simulink model "model"  (R2014a)
(part 5 of 5)

  bus45 : powerlib/Measurements/Load Flow Bus  LConnTagsString=a  ID=bus45  Vbase=220000  Vref=1  Vangle=0  VLF=1  angleLF=0
      settings: AttributesFormatString=|
      | %<ID>
      | %<Vbase>V
      | %<VLF>pu
      | %<angleLF>deg.
      | %<Name>
  bus46 : powerlib/Measurements/Load Flow Bus  LConnTagsString=a  ID=bus46  Vbase=220000  Vref=1  Vangle=0  VLF=1  angleLF=0
      settings: AttributesFormatString=|
      | %<ID>
      | %<Vbase>V
      | %<VLF>pu
      | %<angleLF>deg.
      | %<Name>
  bus47 : powerlib/Measurements/Load Flow Bus  LConnTagsString=a  ID=bus47  Vbase=220000  Vref=1  Vangle=0  VLF=1  angleLF=0
      settings: AttributesFormatString=|
      | %<ID>
      | %<Vbase>V
      | %<VLF>pu
      | %<angleLF>deg.
      | %<Name>
  bus48 : powerlib/Measurements/Load Flow Bus  LConnTagsString=a  ID=bus48  Vbase=220000  Vref=1  Vangle=0  VLF=1  angleLF=0
      settings: AttributesFormatString=|
      | %<ID>
      | %<Vbase>V
      | %<VLF>pu
      | %<angleLF>deg.
      | %<Name>
  bus49 : powerlib/Measurements/Load Flow Bus  LConnTagsString=a  ID=bus49  Vbase=220000  Vref=1  Vangle=0  VLF=1  angleLF=0
      settings: AttributesFormatString=|
      | %<ID>
      | %<Vbase>V
      | %<VLF>pu
      | %<angleLF>deg.
      | %<Name>
  bus5 : powerlib/Measurements/Load Flow Bus  LConnTagsString=a  ID=bus5  Vbase=10000  Vref=1  Vangle=0  VLF=1  angleLF=0
      settings: AttributesFormatString=|
      | %<ID>
      | %<Vbase>V
      | %<VLF>pu
      | %<angleLF>deg.
      | %<Name>
  bus50 : powerlib/Measurements/Load Flow Bus  LConnTagsString=a  ID=bus50  Vbase=220000  Vref=1  Vangle=0  VLF=1  angleLF=0
      settings: AttributesFormatString=|
      | %<ID>
      | %<Vbase>V
      | %<VLF>pu
      | %<angleLF>deg.
      | %<Name>
  bus51 : powerlib/Measurements/Load Flow Bus  LConnTagsString=a  ID=bus51  Vbase=220000  Vref=1  Vangle=0  VLF=1  angleLF=0
      settings: AttributesFormatString=|
      | %<ID>
      | %<Vbase>V
      | %<VLF>pu
      | %<angleLF>deg.
      | %<Name>
  bus52 : powerlib/Measurements/Load Flow Bus  LConnTagsString=a  ID=bus52  Vbase=220000  Vref=1  Vangle=0  VLF=1  angleLF=0
      settings: AttributesFormatString=|
      | %<ID>
      | %<Vbase>V
      | %<VLF>pu
      | %<angleLF>deg.
      | %<Name>
  bus53 : powerlib/Measurements/Load Flow Bus  LConnTagsString=a  ID=bus53  Vbase=220000  Vref=1  Vangle=0  VLF=1  angleLF=0
      settings: AttributesFormatString=|
      | %<ID>
      | %<Vbase>V
      | %<VLF>pu
      | %<angleLF>deg.
      | %<Name>
  bus54 : powerlib/Measurements/Load Flow Bus  LConnTagsString=a  ID=bus54  Vbase=220000  Vref=1  Vangle=0  VLF=1  angleLF=0
      settings: AttributesFormatString=|
      | %<ID>
      | %<Vbase>V
      | %<VLF>pu
      | %<angleLF>deg.
      | %<Name>
  bus55 : powerlib/Measurements/Load Flow Bus  LConnTagsString=a  ID=bus55  Vbase=220000  Vref=1  Vangle=0  VLF=1  angleLF=0
      settings: AttributesFormatString=|
      | %<ID>
      | %<Vbase>V
      | %<VLF>pu
      | %<angleLF>deg.
      | %<Name>
  bus56 : powerlib/Measurements/Load Flow Bus  LConnTagsString=a  ID=bus56  Vbase=220000  Vref=1  Vangle=0  VLF=1  angleLF=0
      settings: AttributesFormatString=|
      | %<ID>
      | %<Vbase>V
      | %<VLF>pu
      | %<angleLF>deg.
      | %<Name>
  bus57 : powerlib/Measurements/Load Flow Bus  LConnTagsString=a  ID=bus57  Vbase=220000  Vref=1  Vangle=0  VLF=1  angleLF=0
      settings: AttributesFormatString=|
      | %<ID>
      | %<Vbase>V
      | %<VLF>pu
      | %<angleLF>deg.
      | %<Name>
  bus58 : powerlib/Measurements/Load Flow Bus  LConnTagsString=a  ID=bus58  Vbase=220000  Vref=1  Vangle=0  VLF=1  angleLF=0
      settings: AttributesFormatString=|
      | %<ID>
      | %<Vbase>V
      | %<VLF>pu
      | %<angleLF>deg.
      | %<Name>
  bus59 : powerlib/Measurements/Load Flow Bus  LConnTagsString=a  ID=bus59  Vbase=220000  Vref=1  Vangle=0  VLF=1  angleLF=0
      settings: AttributesFormatString=|
      | %<ID>
      | %<Vbase>V
      | %<VLF>pu
      | %<angleLF>deg.
      | %<Name>
  bus6 : powerlib/Measurements/Load Flow Bus  LConnTagsString=a  ID=bus6  Vbase=10000  Vref=1  Vangle=0  VLF=1  angleLF=0
      settings: AttributesFormatString=|
      | %<ID>
      | %<Vbase>V
      | %<VLF>pu
      | %<angleLF>deg.
      | %<Name>
  bus60 : powerlib/Measurements/Load Flow Bus  LConnTagsString=a  ID=bus60  Vbase=220000  Vref=1  Vangle=0  VLF=1  angleLF=0
      settings: AttributesFormatString=|
      | %<ID>
      | %<Vbase>V
      | %<VLF>pu
      | %<angleLF>deg.
      | %<Name>
  bus61 : powerlib/Measurements/Load Flow Bus  LConnTagsString=a  ID=bus61  Vbase=220000  Vref=1  Vangle=0  VLF=1  angleLF=0
      settings: AttributesFormatString=|
      | %<ID>
      | %<Vbase>V
      | %<VLF>pu
      | %<angleLF>deg.
      | %<Name>
  bus62 : powerlib/Measurements/Load Flow Bus  LConnTagsString=a  ID=bus62  Vbase=220000  Vref=1  Vangle=0  VLF=1  angleLF=0
      settings: AttributesFormatString=|
      | %<ID>
      | %<Vbase>V
      | %<VLF>pu
      | %<angleLF>deg.
      | %<Name>
  bus63 : powerlib/Measurements/Load Flow Bus  LConnTagsString=a  ID=bus63  Vbase=220000  Vref=1  Vangle=0  VLF=1  angleLF=0
      settings: AttributesFormatString=|
      | %<ID>
      | %<Vbase>V
      | %<VLF>pu
      | %<angleLF>deg.
      | %<Name>
  bus64 : powerlib/Measurements/Load Flow Bus  LConnTagsString=a  ID=bus64  Vbase=220000  Vref=1  Vangle=0  VLF=1  angleLF=0
      settings: AttributesFormatString=|
      | %<ID>
      | %<Vbase>V
      | %<VLF>pu
      | %<angleLF>deg.
      | %<Name>
  bus65 : powerlib/Measurements/Load Flow Bus  LConnTagsString=a  ID=bus65  Vbase=220000  Vref=1  Vangle=0  VLF=1  angleLF=0
      settings: AttributesFormatString=|
      | %<ID>
      | %<Vbase>V
      | %<VLF>pu
      | %<angleLF>deg.
      | %<Name>
  bus66 : powerlib/Measurements/Load Flow Bus  LConnTagsString=a  ID=bus66  Vbase=220000  Vref=1  Vangle=0  VLF=1  angleLF=0
      settings: AttributesFormatString=|
      | %<ID>
      | %<Vbase>V
      | %<VLF>pu
      | %<angleLF>deg.
      | %<Name>
  bus67 : powerlib/Measurements/Load Flow Bus  LConnTagsString=a  ID=bus67  Vbase=220000  Vref=1  Vangle=0  VLF=1  angleLF=0
      settings: AttributesFormatString=|
      | %<ID>
      | %<Vbase>V
      | %<VLF>pu
      | %<angleLF>deg.
      | %<Name>
  bus68 : powerlib/Measurements/Load Flow Bus  LConnTagsString=a  ID=bus68  Vbase=220000  Vref=1  Vangle=0  VLF=1  angleLF=0
      settings: AttributesFormatString=|
      | %<ID>
      | %<Vbase>V
      | %<VLF>pu
      | %<angleLF>deg.
      | %<Name>
  bus69 : powerlib/Measurements/Load Flow Bus  LConnTagsString=a  ID=bus69  Vbase=220000  Vref=1  Vangle=0  VLF=1  angleLF=0
      settings: AttributesFormatString=|
      | %<ID>
      | %<Vbase>V
      | %<VLF>pu
      | %<angleLF>deg.
      | %<Name>
  bus7 : powerlib/Measurements/Load Flow Bus  LConnTagsString=a  ID=bus7  Vbase=10000  Vref=1  Vangle=0  VLF=1  angleLF=0
      settings: AttributesFormatString=|
      | %<ID>
      | %<Vbase>V
      | %<VLF>pu
      | %<angleLF>deg.
      | %<Name>
  bus70 : powerlib/Measurements/Load Flow Bus  LConnTagsString=a  ID=bus70  Vbase=220000  Vref=1  Vangle=0  VLF=1  angleLF=0
      settings: AttributesFormatString=|
      | %<ID>
      | %<Vbase>V
      | %<VLF>pu
      | %<angleLF>deg.
      | %<Name>
  bus71 : powerlib/Measurements/Load Flow Bus  LConnTagsString=a  ID=bus71  Vbase=220000  Vref=1  Vangle=0  VLF=1  angleLF=0
      settings: AttributesFormatString=|
      | %<ID>
      | %<Vbase>V
      | %<VLF>pu
      | %<angleLF>deg.
      | %<Name>
  bus72 : powerlib/Measurements/Load Flow Bus  LConnTagsString=a  ID=bus72  Vbase=220000  Vref=1  Vangle=0  VLF=1  angleLF=0
      settings: AttributesFormatString=|
      | %<ID>
      | %<Vbase>V
      | %<VLF>pu
      | %<angleLF>deg.
      | %<Name>
  bus73 : powerlib/Measurements/Load Flow Bus  LConnTagsString=a  ID=bus73  Vbase=400000  Vref=1  Vangle=0  VLF=1  angleLF=0
      settings: AttributesFormatString=|
      | %<ID>
      | %<Vbase>V
      | %<VLF>pu
      | %<angleLF>deg.
      | %<Name>
  bus74 : powerlib/Measurements/Load Flow Bus  LConnTagsString=a  ID=bus74  Vbase=400000  Vref=1  Vangle=0  VLF=1  angleLF=0
      settings: AttributesFormatString=|
      | %<ID>
      | %<Vbase>V
      | %<VLF>pu
      | %<angleLF>deg.
      | %<Name>
  bus75 : powerlib/Measurements/Load Flow Bus  LConnTagsString=a  ID=bus75  Vbase=400000  Vref=1  Vangle=0  VLF=1  angleLF=0
      settings: AttributesFormatString=|
      | %<ID>
      | %<Vbase>V
      | %<VLF>pu
      | %<angleLF>deg.
      | %<Name>
  bus76 : powerlib/Measurements/Load Flow Bus  LConnTagsString=a  ID=bus76  Vbase=400000  Vref=1  Vangle=0  VLF=1  angleLF=0
      settings: AttributesFormatString=|
      | %<ID>
      | %<Vbase>V
      | %<VLF>pu
      | %<angleLF>deg.
      | %<Name>
  bus77 : powerlib/Measurements/Load Flow Bus  LConnTagsString=a  ID=bus77  Vbase=400000  Vref=1  Vangle=0  VLF=1  angleLF=0
      settings: AttributesFormatString=|
      | %<ID>
      | %<Vbase>V
      | %<VLF>pu
      | %<angleLF>deg.
      | %<Name>
  bus78 : powerlib/Measurements/Load Flow Bus  LConnTagsString=a  ID=bus78  Vbase=400000  Vref=1  Vangle=0  VLF=1  angleLF=0
      settings: AttributesFormatString=|
      | %<ID>
      | %<Vbase>V
      | %<VLF>pu
      | %<angleLF>deg.
      | %<Name>
  bus79 : powerlib/Measurements/Load Flow Bus  LConnTagsString=a  ID=bus79  Vbase=400000  Vref=1  Vangle=0  VLF=1  angleLF=0
      settings: AttributesFormatString=|
      | %<ID>
      | %<Vbase>V
      | %<VLF>pu
      | %<angleLF>deg.
      | %<Name>
  bus8 : powerlib/Measurements/Load Flow Bus  LConnTagsString=a  ID=bus8  Vbase=10000  Vref=1  Vangle=0  VLF=1  angleLF=0
      settings: AttributesFormatString=|
      | %<ID>
      | %<Vbase>V
      | %<VLF>pu
      | %<angleLF>deg.
      | %<Name>
  bus80 : powerlib/Measurements/Load Flow Bus  LConnTagsString=a  ID=bus80  Vbase=400000  Vref=1  Vangle=0  VLF=1  angleLF=0
      settings: AttributesFormatString=|
      | %<ID>
      | %<Vbase>V
      | %<VLF>pu
      | %<angleLF>deg.
      | %<Name>
  bus81 : powerlib/Measurements/Load Flow Bus  LConnTagsString=a  ID=bus81  Vbase=400000  Vref=1  Vangle=0  VLF=1  angleLF=0
      settings: AttributesFormatString=|
      | %<ID>
      | %<Vbase>V
      | %<VLF>pu
      | %<angleLF>deg.
      | %<Name>
  bus82 : powerlib/Measurements/Load Flow Bus  LConnTagsString=a  ID=bus82  Vbase=400000  Vref=1  Vangle=0  VLF=1  angleLF=0
      settings: AttributesFormatString=|
      | %<ID>
      | %<Vbase>V
      | %<VLF>pu
      | %<angleLF>deg.
      | %<Name>
  bus83 : powerlib/Measurements/Load Flow Bus  LConnTagsString=a  ID=bus83  Vbase=400000  Vref=1  Vangle=0  VLF=1  angleLF=0
      settings: AttributesFormatString=|
      | %<ID>
      | %<Vbase>V
      | %<VLF>pu
      | %<angleLF>deg.
      | %<Name>
  bus84 : powerlib/Measurements/Load Flow Bus  LConnTagsString=a  ID=bus84  Vbase=400000  Vref=1  Vangle=0  VLF=1  angleLF=0
      settings: AttributesFormatString=|
      | %<ID>
      | %<Vbase>V
      | %<VLF>pu
      | %<angleLF>deg.
      | %<Name>
  bus85 : powerlib/Measurements/Load Flow Bus  LConnTagsString=a  ID=bus85  Vbase=400000  Vref=1  Vangle=0  VLF=1  angleLF=0
      settings: AttributesFormatString=|
      | %<ID>
      | %<Vbase>V
      | %<VLF>pu
      | %<angleLF>deg.
      | %<Name>
  bus86 : powerlib/Measurements/Load Flow Bus  LConnTagsString=a  ID=bus86  Vbase=400000  Vref=1  Vangle=0  VLF=1  angleLF=0
      settings: AttributesFormatString=|
      | %<ID>
      | %<Vbase>V
      | %<VLF>pu
      | %<angleLF>deg.
      | %<Name>
  bus87 : powerlib/Measurements/Load Flow Bus  LConnTagsString=a  ID=bus87  Vbase=400000  Vref=1  Vangle=0  VLF=1  angleLF=0
      settings: AttributesFormatString=|
      | %<ID>
      | %<Vbase>V
      | %<VLF>pu
      | %<angleLF>deg.
      | %<Name>
  bus88 : powerlib/Measurements/Load Flow Bus  LConnTagsString=a  ID=bus88  Vbase=400000  Vref=1  Vangle=0  VLF=1  angleLF=0
      settings: AttributesFormatString=|
      | %<ID>
      | %<Vbase>V
      | %<VLF>pu
      | %<angleLF>deg.
      | %<Name>
  bus89 : powerlib/Measurements/Load Flow Bus  LConnTagsString=a  ID=bus89  Vbase=400000  Vref=1  Vangle=0  VLF=1  angleLF=0
      settings: AttributesFormatString=|
      | %<ID>
      | %<Vbase>V
      | %<VLF>pu
      | %<angleLF>deg.
      | %<Name>
  bus9 : powerlib/Measurements/Load Flow Bus  LConnTagsString=a  ID=bus9  Vbase=10000  Vref=1  Vangle=0  VLF=1  angleLF=0
      settings: AttributesFormatString=|
      | %<ID>
      | %<Vbase>V
      | %<VLF>pu
      | %<angleLF>deg.
      | %<Name>
  bus90 : powerlib/Measurements/Load Flow Bus  LConnTagsString=a  ID=bus90  Vbase=400000  Vref=1  Vangle=0  VLF=1  angleLF=0
      settings: AttributesFormatString=|
      | %<ID>
      | %<Vbase>V
      | %<VLF>pu
      | %<angleLF>deg.
      | %<Name>
  bus91 : powerlib/Measurements/Load Flow Bus  LConnTagsString=a  ID=bus91  Vbase=400000  Vref=1  Vangle=0  VLF=1  angleLF=0
      settings: AttributesFormatString=|
      | %<ID>
      | %<Vbase>V
      | %<VLF>pu
      | %<angleLF>deg.
      | %<Name>
  bus92 : powerlib/Measurements/Load Flow Bus  LConnTagsString=a  ID=bus92  Vbase=400000  Vref=1  Vangle=0  VLF=1  angleLF=0
      settings: AttributesFormatString=|
      | %<ID>
      | %<Vbase>V
      | %<VLF>pu
      | %<angleLF>deg.
      | %<Name>
  bus93 : powerlib/Measurements/Load Flow Bus  LConnTagsString=a  ID=bus93  Vbase=400000  Vref=1  Vangle=0  VLF=1  angleLF=0
      settings: AttributesFormatString=|
      | %<ID>
      | %<Vbase>V
      | %<VLF>pu
      | %<angleLF>deg.
      | %<Name>
  bus94 : powerlib/Measurements/Load Flow Bus  LConnTagsString=a  ID=bus94  Vbase=400000  Vref=1  Vangle=0  VLF=1  angleLF=0
      settings: AttributesFormatString=|
      | %<ID>
      | %<Vbase>V
      | %<VLF>pu
      | %<angleLF>deg.
      | %<Name>
  bus95 : powerlib/Measurements/Load Flow Bus  LConnTagsString=a  ID=bus95  Vbase=400000  Vref=1  Vangle=0  VLF=1  angleLF=0
      settings: AttributesFormatString=|
      | %<ID>
      | %<Vbase>V
      | %<VLF>pu
      | %<angleLF>deg.
      | %<Name>
  bus96 : powerlib/Measurements/Load Flow Bus  LConnTagsString=a  ID=bus96  Vbase=400000  Vref=1  Vangle=0  VLF=1  angleLF=0
      settings: AttributesFormatString=|
      | %<ID>
      | %<Vbase>V
      | %<VLF>pu
      | %<angleLF>deg.
      | %<Name>
  bus97 : powerlib/Measurements/Load Flow Bus  LConnTagsString=a  ID=bus97  Vbase=400000  Vref=1  Vangle=0  VLF=1  angleLF=0
      settings: AttributesFormatString=|
      | %<ID>
      | %<Vbase>V
      | %<VLF>pu
      | %<angleLF>deg.
      | %<Name>
  bus98 : powerlib/Measurements/Load Flow Bus  LConnTagsString=a  ID=bus98  Vbase=400000  Vref=1  Vangle=0  VLF=1  angleLF=0
      settings: AttributesFormatString=|
      | %<ID>
      | %<Vbase>V
      | %<VLF>pu
      | %<angleLF>deg.
      | %<Name>
  bus99 : powerlib/Measurements/Load Flow Bus  LConnTagsString=a  ID=bus99  Vbase=400000  Vref=1  Vangle=0  VLF=1  angleLF=0
      settings: AttributesFormatString=|
      | %<ID>
      | %<Vbase>V
      | %<VLF>pu
      | %<angleLF>deg.
      | %<Name>
  powergui : powerlib/powergui  Priority=1  SimulationMode=Continuous  SolverType=Tustin  SampleTime=50e-6  frequency=60  SPID=off  DisableSnubberDevices=off  DisableRonSwitches=off  DisableVfSwitches=off  SwTol=0  Interpol=off  DisplayEquations=off  Ts=0  methode=off  frequencyindice=60  Pbase=100e6  ErrMax=1e-4  Iterations=50  UnitsV=kV  UnitsW=MW  FunctionMessages=off  echomessages=off  HookPort=off  EnableUseOfTLC=off  x0status=blocks  RestoreLinks=warning  ResistiveCurrentMeasurement=off  Frange=[0:2:500]  Ylog=off  Xlog=on  ShowGrid=off  save=off  variable=ZData  structure=0  ZoomFFT=off  StartTime=0.0  cycles=1  DisplayStyle=1  fundamental=60  FreqAxis=off  MaxFrequency=1000  frequencyindicesteady=1  RmsSteady=1  display=off
  Ötztal___Zirl_CN_147563007_110000_CN_100404264_110000 : powerlib/Elements/Distributed Parameters Line  Phases=3  Frequency=60  Resistance=[0.01273 0.3864]  Inductance="[0.9337e-3  4.1264e-3]"  Capacitance=[12.74e-9 7.751e-9]  Length=100  x1=[0 0 0 0; 0.0001244 0 0 0; 0.0002488 0 0 0; 0.0003733 0 0 0; 0.0004977 0 0 0; 0.0006221 0 0 0]  x2=[0 0 0 0; 0.0001244 0 0 0; 0.0002488 0 0 0; 0.0003733 0 0 0; 0.0004977 0 0 0; 0.0006221 0 0 0]  x3=[0 0 0 0; 0.0001244 0 0 0; 0.0002488 0 0 0; 0.0003733 0 0 0; 0.0004977 0 0 0; 0.0006221 0 0 0]  x4=[0 0 0 0; 0.0001244 0 0 0; 0.0002488 0 0 0; 0.0003733 0 0 0; 0.0004977 0 0 0; 0.0006221 0 0 0]  x5=0  V1=ones(3,3)  V2=ones(3,3)  I1=ones(3,3)  I2=ones(3,3)  nHarmo=1  Measurements=None
  connections:
  T_48374400__/LConn1 -- _CN_48374400_10000_CN_46584322_10000/LConn1
  T_48374400__/LConn2 -- _CN_48374400_10000_CN_46584322_10000/LConn2
  _CN_48374400_10000_CN_46584322_10000/LConn3 -- T_48374400__/LConn3 -- bus1/LConn1
  T_46584322__/LConn1 -- _CN_48374400_10000_CN_46584322_10000/RConn1
  T_46584322__/LConn2 -- _CN_48374400_10000_CN_46584322_10000/RConn2
  _CN_48374400_10000_CN_46584322_10000/RConn3 -- T_46584322__/LConn3 -- bus2/LConn1
  _CN_209067396_10000_CN_30621843_10000/LConn1 -- T_209067396__/LConn1 -- _CN_209067396_10000_CN_30622639_10000/LConn1
  _CN_209067396_10000_CN_30621843_10000/LConn2 -- T_209067396__/LConn2 -- _CN_209067396_10000_CN_30622639_10000/LConn2
  _CN_209067396_10000_CN_30621843_10000/LConn3 -- T_209067396__/LConn3 -- _CN_209067396_10000_CN_30622639_10000/LConn3 -- bus3/LConn1
  T_30621843__/LConn1 -- _CN_209067396_10000_CN_30621843_10000/RConn1
  T_30621843__/LConn2 -- _CN_209067396_10000_CN_30621843_10000/RConn2
  _CN_209067396_10000_CN_30621843_10000/RConn3 -- T_30621843__/LConn3 -- bus4/LConn1
  _CN_209067396_10000_CN_30622639_10000/RConn1 -- T_30622639__/LConn1 -- _CN_30622639_10000_CN_37036252_10000/LConn1
  _CN_209067396_10000_CN_30622639_10000/RConn2 -- T_30622639__/LConn2 -- _CN_30622639_10000_CN_37036252_10000/LConn2
  _CN_209067396_10000_CN_30622639_10000/RConn3 -- T_30622639__/LConn3 -- _CN_30622639_10000_CN_37036252_10000/LConn3 -- bus5/LConn1
  T_207939980__/LConn1 -- 110kV_CN_207939980_10000_CN_97334781_10000/LConn1
  T_207939980__/LConn2 -- 110kV_CN_207939980_10000_CN_97334781_10000/LConn2
  110kV_CN_207939980_10000_CN_97334781_10000/LConn3 -- T_207939980__/LConn3 -- bus6/LConn1
  110kV_CN_207939980_10000_CN_97334781_10000/RConn1 -- T_97334781__/RConn1 -- _CN_97334822_10000_CN_97334781_10000/LConn1 -- _CN_97418808_10000_CN_97334781_10000/LConn1 -- _CN_176828096_10000_CN_97334781_10000/LConn1 -- L_97334781/LConn1 -- 110kV_CN_176819478_10000_CN_97334781_10000/LConn1
  110kV_CN_207939980_10000_CN_97334781_10000/RConn2 -- T_97334781__/RConn2 -- _CN_97334822_10000_CN_97334781_10000/LConn2 -- _CN_97418808_10000_CN_97334781_10000/LConn2 -- _CN_176828096_10000_CN_97334781_10000/LConn2 -- L_97334781/LConn2 -- 110kV_CN_176819478_10000_CN_97334781_10000/LConn2
  110kV_CN_207939980_10000_CN_97334781_10000/RConn3 -- T_97334781__/RConn3 -- _CN_97334822_10000_CN_97334781_10000/LConn3 -- _CN_97418808_10000_CN_97334781_10000/LConn3 -- _CN_176828096_10000_CN_97334781_10000/LConn3 -- L_97334781/LConn3 -- bus7/LConn1 -- 110kV_CN_176819478_10000_CN_97334781_10000/LConn3
  T_176819478__Statie_de_transformare_110kV_20kV/LConn1 -- 110kV_CN_176819478_10000_CN_97334781_10000/RConn1
  T_176819478__Statie_de_transformare_110kV_20kV/LConn2 -- 110kV_CN_176819478_10000_CN_97334781_10000/RConn2
  110kV_CN_176819478_10000_CN_97334781_10000/RConn3 -- T_176819478__Statie_de_transformare_110kV_20kV/LConn3 -- bus8/LConn1
  _CN_234876695_10000_CN_97418808_10000/LConn1 -- T_234876695__/RConn4 -- L_234876695/LConn1
  _CN_234876695_10000_CN_97418808_10000/LConn2 -- T_234876695__/RConn5 -- L_234876695/LConn2
  _CN_234876695_10000_CN_97418808_10000/LConn3 -- T_234876695__/RConn6 -- L_234876695/LConn3 -- bus9/LConn1
  _CN_234876695_10000_CN_97418808_10000/RConn1 -- T_97418808__/LConn1 -- _CN_97418808_10000_CN_97334781_10000/RConn1
  _CN_234876695_10000_CN_97418808_10000/RConn2 -- T_97418808__/LConn2 -- _CN_97418808_10000_CN_97334781_10000/RConn2
  _CN_234876695_10000_CN_97418808_10000/RConn3 -- T_97418808__/LConn3 -- _CN_97418808_10000_CN_97334781_10000/RConn3 -- bus10/LConn1
  T_204932122__/LConn1 -- _CN_204932122_10000_CN_198333274_10000/LConn1
  T_204932122__/LConn2 -- _CN_204932122_10000_CN_198333274_10000/LConn2
  _CN_204932122_10000_CN_198333274_10000/LConn3 -- T_204932122__/LConn3 -- bus11/LConn1
  T_198333274__/LConn1 -- _CN_204932122_10000_CN_198333274_10000/RConn1
  T_198333274__/LConn2 -- _CN_204932122_10000_CN_198333274_10000/RConn2
  _CN_204932122_10000_CN_198333274_10000/RConn3 -- T_198333274__/LConn3 -- bus12/LConn1
  T_97334822__/LConn1 -- _CN_97334822_10000_CN_97334781_10000/RConn1
  T_97334822__/LConn2 -- _CN_97334822_10000_CN_97334781_10000/RConn2
  _CN_97334822_10000_CN_97334781_10000/RConn3 -- T_97334822__/LConn3 -- bus13/LConn1
  _CN_28251692_10000_CN_30618879_10000/LConn1 -- T_28251692__/RConn1 -- L_28251692/LConn1
  _CN_28251692_10000_CN_30618879_10000/LConn2 -- T_28251692__/RConn2 -- L_28251692/LConn2
  _CN_28251692_10000_CN_30618879_10000/LConn3 -- T_28251692__/RConn3 -- L_28251692/LConn3 -- bus14/LConn1
  G_30618879_CET_Vest/RConn1 -- _CN_28251692_10000_CN_30618879_10000/RConn1
  G_30618879_CET_Vest/RConn2 -- _CN_28251692_10000_CN_30618879_10000/RConn2
  _CN_28251692_10000_CN_30618879_10000/RConn3 -- G_30618879_CET_Vest/RConn3 -- bus15/LConn1
  _CN_30622639_10000_CN_37036252_10000/RConn1 -- T_37036252__/LConn1 -- _CN_37036252_10000_CN_29975403_10000/LConn1
  _CN_30622639_10000_CN_37036252_10000/RConn2 -- T_37036252__/LConn2 -- _CN_37036252_10000_CN_29975403_10000/LConn2
  _CN_30622639_10000_CN_37036252_10000/RConn3 -- T_37036252__/LConn3 -- _CN_37036252_10000_CN_29975403_10000/LConn3 -- bus16/LConn1
  _CN_176828096_10000_CN_97334781_10000/RConn1 -- T_176828096__/LConn1 -- _CN_176828096_10000_CN_235313249_10000/LConn1
  _CN_176828096_10000_CN_97334781_10000/RConn2 -- T_176828096__/LConn2 -- _CN_176828096_10000_CN_235313249_10000/LConn2
  _CN_176828096_10000_CN_97334781_10000/RConn3 -- T_176828096__/LConn3 -- _CN_176828096_10000_CN_235313249_10000/LConn3 -- bus17/LConn1
  T_235313249__/LConn1 -- _CN_176828096_10000_CN_235313249_10000/RConn1
  T_235313249__/LConn2 -- _CN_176828096_10000_CN_235313249_10000/RConn2
  _CN_176828096_10000_CN_235313249_10000/RConn3 -- T_235313249__/LConn3 -- bus18/LConn1
  T_29975403__/LConn1 -- _CN_37036252_10000_CN_29975403_10000/RConn1
  T_29975403__/LConn2 -- _CN_37036252_10000_CN_29975403_10000/RConn2
  _CN_37036252_10000_CN_29975403_10000/RConn3 -- T_29975403__/LConn3 -- bus19/LConn1
  T_89071477__/LConn1 -- _CN_89071477_10000_CN_46269303_10000/LConn1
  T_89071477__/LConn2 -- _CN_89071477_10000_CN_46269303_10000/LConn2
  _CN_89071477_10000_CN_46269303_10000/LConn3 -- T_89071477__/LConn3 -- bus20/LConn1
  T_46269303__/LConn1 -- _CN_89071477_10000_CN_46269303_10000/RConn1
  T_46269303__/LConn2 -- _CN_89071477_10000_CN_46269303_10000/RConn2
  _CN_89071477_10000_CN_46269303_10000/RConn3 -- T_46269303__/LConn3 -- bus21/LConn1
  T_278910976__/LConn1 -- _CN_278910976_220000_CN_199657993_220000/LConn1
  T_278910976__/LConn2 -- _CN_278910976_220000_CN_199657993_220000/LConn2
  _CN_278910976_220000_CN_199657993_220000/LConn3 -- T_278910976__/LConn3 -- bus22/LConn1
  T_199657993__/LConn1 -- _CN_278910976_220000_CN_199657993_220000/RConn1
  T_199657993__/LConn2 -- _CN_278910976_220000_CN_199657993_220000/RConn2
  _CN_278910976_220000_CN_199657993_220000/RConn3 -- T_199657993__/LConn3 -- bus23/LConn1
  T_208744453__/LConn1 -- _CN_208744453_220000_CN_228718321_220000/LConn1
  T_208744453__/LConn2 -- _CN_208744453_220000_CN_228718321_220000/LConn2
  _CN_208744453_220000_CN_228718321_220000/LConn3 -- T_208744453__/LConn3 -- bus24/LConn1
  _CN_208744453_220000_CN_228718321_220000/RConn1 -- T_228718321__/RConn1 -- _CN_208263464_220000_CN_228718321_220000/LConn1 -- L_228718321/LConn1
  _CN_208744453_220000_CN_228718321_220000/RConn2 -- T_228718321__/RConn2 -- _CN_208263464_220000_CN_228718321_220000/LConn2 -- L_228718321/LConn2
  _CN_208744453_220000_CN_228718321_220000/RConn3 -- T_228718321__/RConn3 -- _CN_208263464_220000_CN_228718321_220000/LConn3 -- L_228718321/LConn3 -- bus25/LConn1
  T_198276673__/LConn1 -- _CN_198276673_220000_CN_202461729_220000/LConn1
  T_198276673__/LConn2 -- _CN_198276673_220000_CN_202461729_220000/LConn2
  _CN_198276673_220000_CN_202461729_220000/LConn3 -- T_198276673__/LConn3 -- bus26/LConn1
  _CN_198276673_220000_CN_202461729_220000/RConn1 -- T_202461729__/LConn1 -- _CN_202948507_220000_CN_202461729_220000/LConn1
  _CN_198276673_220000_CN_202461729_220000/RConn2 -- T_202461729__/LConn2 -- _CN_202948507_220000_CN_202461729_220000/LConn2
  _CN_198276673_220000_CN_202461729_220000/RConn3 -- T_202461729__/LConn3 -- _CN_202948507_220000_CN_202461729_220000/LConn3 -- bus27/LConn1
  _CN_98111242_220000_CN_196654384_220000/LConn1 -- T_98111242__/LConn1 -- _CN_98111242_220000_CN_208263479_220000/LConn1 -- _CN_98111242_220000_CN_198283094_220000/LConn1 -- _CN_98111242_220000_CN_234876695_220000/LConn1 -- _CN_98111242_220000_CN_196654364_220000/LConn1 -- _CN_98111242_220000_CN_196654362_220000/LConn1 -- _CN_98111242_220000_CN_88174437_220000/LConn1
  _CN_98111242_220000_CN_196654384_220000/LConn2 -- T_98111242__/LConn2 -- _CN_98111242_220000_CN_208263479_220000/LConn2 -- _CN_98111242_220000_CN_198283094_220000/LConn2 -- _CN_98111242_220000_CN_234876695_220000/LConn2 -- _CN_98111242_220000_CN_196654364_220000/LConn2 -- _CN_98111242_220000_CN_196654362_220000/LConn2 -- _CN_98111242_220000_CN_88174437_220000/LConn2
  _CN_98111242_220000_CN_196654384_220000/LConn3 -- T_98111242__/LConn3 -- _CN_98111242_220000_CN_208263479_220000/LConn3 -- _CN_98111242_220000_CN_198283094_220000/LConn3 -- _CN_98111242_220000_CN_234876695_220000/LConn3 -- _CN_98111242_220000_CN_196654364_220000/LConn3 -- _CN_98111242_220000_CN_196654362_220000/LConn3 -- _CN_98111242_220000_CN_88174437_220000/LConn3 -- bus28/LConn1
  T_196654384__/LConn1 -- _CN_98111242_220000_CN_196654384_220000/RConn1
  T_196654384__/LConn2 -- _CN_98111242_220000_CN_196654384_220000/RConn2
  _CN_98111242_220000_CN_196654384_220000/RConn3 -- T_196654384__/LConn3 -- bus29/LConn1
  T_208263479__/LConn1 -- _CN_98111242_220000_CN_208263479_220000/RConn1
  T_208263479__/LConn2 -- _CN_98111242_220000_CN_208263479_220000/RConn2
  _CN_98111242_220000_CN_208263479_220000/RConn3 -- T_208263479__/LConn3 -- bus30/LConn1
  T_198283094__/LConn1 -- _CN_98111242_220000_CN_198283094_220000/RConn1
  T_198283094__/LConn2 -- _CN_98111242_220000_CN_198283094_220000/RConn2
  _CN_98111242_220000_CN_198283094_220000/RConn3 -- T_198283094__/LConn3 -- bus31/LConn1
  _CN_98111242_220000_CN_234876695_220000/RConn1 -- T_234876695__/RConn1 -- _CN_234876695_220000_CN_97334781_220000/LConn1
  _CN_98111242_220000_CN_234876695_220000/RConn2 -- T_234876695__/RConn2 -- _CN_234876695_220000_CN_97334781_220000/LConn2
  _CN_98111242_220000_CN_234876695_220000/RConn3 -- T_234876695__/RConn3 -- _CN_234876695_220000_CN_97334781_220000/LConn3 -- bus32/LConn1
  T_196654364__/LConn1 -- _CN_98111242_220000_CN_196654364_220000/RConn1
  T_196654364__/LConn2 -- _CN_98111242_220000_CN_196654364_220000/RConn2
  _CN_98111242_220000_CN_196654364_220000/RConn3 -- T_196654364__/LConn3 -- bus33/LConn1
  T_196654362__/LConn1 -- _CN_98111242_220000_CN_196654362_220000/RConn1
  T_196654362__/LConn2 -- _CN_98111242_220000_CN_196654362_220000/RConn2
  _CN_98111242_220000_CN_196654362_220000/RConn3 -- T_196654362__/LConn3 -- bus34/LConn1
  _CN_98111242_220000_CN_88174437_220000/RConn1 -- G_88174437_Termocentrala_Mintia/RConn1 -- _CN_196654321_400000_CN_88174437_220000/LConn1 -- _CN_71212865_220000_CN_88174437_220000/LConn1 -- _CN_101158766_400000_CN_88174437_220000/LConn1
  _CN_98111242_220000_CN_88174437_220000/RConn2 -- G_88174437_Termocentrala_Mintia/RConn2 -- _CN_196654321_400000_CN_88174437_220000/LConn2 -- _CN_71212865_220000_CN_88174437_220000/LConn2 -- _CN_101158766_400000_CN_88174437_220000/LConn2
  _CN_98111242_220000_CN_88174437_220000/RConn3 -- G_88174437_Termocentrala_Mintia/RConn3 -- _CN_196654321_400000_CN_88174437_220000/LConn3 -- bus35/LConn1 -- _CN_71212865_220000_CN_88174437_220000/LConn3 -- _CN_101158766_400000_CN_88174437_220000/LConn3
  _CN_234876695_220000_CN_97334781_220000/RConn1 -- T_97334781__/LConn1 -- _CN_97334781_220000_CN_266629200_220000/LConn1
  _CN_234876695_220000_CN_97334781_220000/RConn2 -- T_97334781__/LConn2 -- _CN_97334781_220000_CN_266629200_220000/LConn2
  _CN_234876695_220000_CN_97334781_220000/RConn3 -- T_97334781__/LConn3 -- _CN_97334781_220000_CN_266629200_220000/LConn3 -- bus36/LConn1
  T_108198802__/LConn1 -- _CN_108198802_220000_CN_108198777_220000/LConn1
  T_108198802__/LConn2 -- _CN_108198802_220000_CN_108198777_220000/LConn2
  _CN_108198802_220000_CN_108198777_220000/LConn3 -- T_108198802__/LConn3 -- bus37/LConn1
  T_108198777__/LConn1 -- _CN_108198802_220000_CN_108198777_220000/RConn1
  T_108198777__/LConn2 -- _CN_108198802_220000_CN_108198777_220000/RConn2
  _CN_108198802_220000_CN_108198777_220000/RConn3 -- T_108198777__/LConn3 -- bus38/LConn1
  T_30621463__/LConn1 -- _CN_30621463_220000_CN_198310955_220000/LConn1
  T_30621463__/LConn2 -- _CN_30621463_220000_CN_198310955_220000/LConn2
  _CN_30621463_220000_CN_198310955_220000/LConn3 -- T_30621463__/LConn3 -- bus39/LConn1
  T_198310955__/LConn1 -- _CN_30621463_220000_CN_198310955_220000/RConn1
  T_198310955__/LConn2 -- _CN_30621463_220000_CN_198310955_220000/RConn2
  _CN_30621463_220000_CN_198310955_220000/RConn3 -- T_198310955__/LConn3 -- bus40/LConn1
  _CN_196672665_220000_CN_196672685_220000/LConn1 -- T_196672665__/RConn1 -- _CN_196672665_220000_CN_88174813_220000/LConn1 -- L_196672665/LConn1
  _CN_196672665_220000_CN_196672685_220000/LConn2 -- T_196672665__/RConn2 -- _CN_196672665_220000_CN_88174813_220000/LConn2 -- L_196672665/LConn2
  _CN_196672665_220000_CN_196672685_220000/LConn3 -- T_196672665__/RConn3 -- _CN_196672665_220000_CN_88174813_220000/LConn3 -- L_196672665/LConn3 -- bus41/LConn1
  _CN_196672665_220000_CN_196672685_220000/RConn1 -- T_196672685__/RConn1 -- L_196672685/LConn1
  _CN_196672665_220000_CN_196672685_220000/RConn2 -- T_196672685__/RConn2 -- L_196672685/LConn2
  _CN_196672665_220000_CN_196672685_220000/RConn3 -- T_196672685__/RConn3 -- L_196672685/LConn3 -- bus42/LConn1
  G_88174813_Galați_Power_Station/RConn1 -- _CN_196672665_220000_CN_88174813_220000/RConn1
  G_88174813_Galați_Power_Station/RConn2 -- _CN_196672665_220000_CN_88174813_220000/RConn2
  _CN_196672665_220000_CN_88174813_220000/RConn3 -- G_88174813_Galați_Power_Station/RConn3 -- bus43/LConn1
  _CN_202948507_220000_CN_202461729_220000/RConn1 -- T_202948507__/RConn1 -- L_202948507/LConn1
  _CN_202948507_220000_CN_202461729_220000/RConn2 -- T_202948507__/RConn2 -- L_202948507/LConn2
  _CN_202948507_220000_CN_202461729_220000/RConn3 -- T_202948507__/RConn3 -- L_202948507/LConn3 -- bus44/LConn1
  _CN_210609562_220000_CN_208294493_220000/LConn1 -- T_210609562__/LConn1 -- _CN_210609562_220000_CN_205384220_220000/LConn1
  _CN_210609562_220000_CN_208294493_220000/LConn2 -- T_210609562__/LConn2 -- _CN_210609562_220000_CN_205384220_220000/LConn2
  _CN_210609562_220000_CN_208294493_220000/LConn3 -- T_210609562__/LConn3 -- _CN_210609562_220000_CN_205384220_220000/LConn3 -- bus45/LConn1
  T_208294493__/LConn1 -- _CN_210609562_220000_CN_208294493_220000/RConn1
  T_208294493__/LConn2 -- _CN_210609562_220000_CN_208294493_220000/RConn2
  _CN_210609562_220000_CN_208294493_220000/RConn3 -- T_208294493__/LConn3 -- bus46/LConn1
  _CN_210609562_220000_CN_205384220_220000/RConn1 -- T_205384220__/RConn1 -- _CN_97872423_220000_CN_205384220_220000/LConn1 -- L_205384220/LConn1
  _CN_210609562_220000_CN_205384220_220000/RConn2 -- T_205384220__/RConn2 -- _CN_97872423_220000_CN_205384220_220000/LConn2 -- L_205384220/LConn2
  _CN_210609562_220000_CN_205384220_220000/RConn3 -- T_205384220__/RConn3 -- _CN_97872423_220000_CN_205384220_220000/LConn3 -- L_205384220/LConn3 -- bus47/LConn1
  _CN_198777633_220000_CN_223680127_220000/LConn1 -- T_198777633__/RConn1 -- _CN_198777633_220000_CN_421929873_220000/LConn1 -- _CN_198777633_220000_CN_198777681_220000/LConn1 -- L_198777633/LConn1
  _CN_198777633_220000_CN_223680127_220000/LConn2 -- T_198777633__/RConn2 -- _CN_198777633_220000_CN_421929873_220000/LConn2 -- _CN_198777633_220000_CN_198777681_220000/LConn2 -- L_198777633/LConn2
  _CN_198777633_220000_CN_223680127_220000/LConn3 -- T_198777633__/RConn3 -- _CN_198777633_220000_CN_421929873_220000/LConn3 -- _CN_198777633_220000_CN_198777681_220000/LConn3 -- L_198777633/LConn3 -- bus48/LConn1
  T_223680127__/LConn1 -- _CN_198777633_220000_CN_223680127_220000/RConn1
  T_223680127__/LConn2 -- _CN_198777633_220000_CN_223680127_220000/RConn2
  _CN_198777633_220000_CN_223680127_220000/RConn3 -- T_223680127__/LConn3 -- bus49/LConn1
  G_421929873_/RConn1 -- _CN_198777633_220000_CN_421929873_220000/RConn1
  G_421929873_/RConn2 -- _CN_198777633_220000_CN_421929873_220000/RConn2
  _CN_198777633_220000_CN_421929873_220000/RConn3 -- G_421929873_/RConn3 -- bus50/LConn1
  _CN_198777633_220000_CN_198777681_220000/RConn1 -- T_198777681__/LConn1 -- _CN_198777681_220000_CN_182886368_220000/LConn1
  _CN_198777633_220000_CN_198777681_220000/RConn2 -- T_198777681__/LConn2 -- _CN_198777681_220000_CN_182886368_220000/LConn2
  _CN_198777633_220000_CN_198777681_220000/RConn3 -- T_198777681__/LConn3 -- _CN_198777681_220000_CN_182886368_220000/LConn3 -- bus51/LConn1
  _CN_103213478_220000_CN_182886368_220000/LConn1 -- T_103213478__/LConn1 -- Linie_electrică_de_înaltă_tensiune_de_220_kV_CN_103213478_220000_CN_23575521_220000/LConn1 -- Linie_electrică_de_înaltă_tensiune_de_220_kV_CN_103213478_220000_CN_74348980_220000/LConn1
  _CN_103213478_220000_CN_182886368_220000/LConn2 -- T_103213478__/LConn2 -- Linie_electrică_de_înaltă_tensiune_de_220_kV_CN_103213478_220000_CN_23575521_220000/LConn2 -- Linie_electrică_de_înaltă_tensiune_de_220_kV_CN_103213478_220000_CN_74348980_220000/LConn2
  _CN_103213478_220000_CN_182886368_220000/LConn3 -- T_103213478__/LConn3 -- Linie_electrică_de_înaltă_tensiune_de_220_kV_CN_103213478_220000_CN_23575521_220000/LConn3 -- Linie_electrică_de_înaltă_tensiune_de_220_kV_CN_103213478_220000_CN_74348980_220000/LConn3 -- bus52/LConn1
  _CN_103213478_220000_CN_182886368_220000/RConn1 -- T_182886368__/LConn1 -- _CN_198777681_220000_CN_182886368_220000/RConn1
  _CN_103213478_220000_CN_182886368_220000/RConn2 -- T_182886368__/LConn2 -- _CN_198777681_220000_CN_182886368_220000/RConn2
  _CN_103213478_220000_CN_182886368_220000/RConn3 -- T_182886368__/LConn3 -- _CN_198777681_220000_CN_182886368_220000/RConn3 -- bus53/LConn1
  Linie_electrică_de_înaltă_tensiune_de_220_kV_CN_103213478_220000_CN_23575521_220000/RConn1 -- T_23575521__/RConn1 -- L_23575521/LConn1
  Linie_electrică_de_înaltă_tensiune_de_220_kV_CN_103213478_220000_CN_23575521_220000/RConn2 -- T_23575521__/RConn2 -- L_23575521/LConn2
  Linie_electrică_de_înaltă_tensiune_de_220_kV_CN_103213478_220000_CN_23575521_220000/RConn3 -- T_23575521__/RConn3 -- L_23575521/LConn3 -- bus54/LConn1
  T_74348980__/LConn1 -- Linie_electrică_de_înaltă_tensiune_de_220_kV_CN_103213478_220000_CN_74348980_220000/RConn1
  T_74348980__/LConn2 -- Linie_electrică_de_înaltă_tensiune_de_220_kV_CN_103213478_220000_CN_74348980_220000/RConn2
  Linie_electrică_de_înaltă_tensiune_de_220_kV_CN_103213478_220000_CN_74348980_220000/RConn3 -- T_74348980__/LConn3 -- bus55/LConn1
  T_97872423__/LConn1 -- _CN_97872423_220000_CN_205384220_220000/RConn1
  T_97872423__/LConn2 -- _CN_97872423_220000_CN_205384220_220000/RConn2
  _CN_97872423_220000_CN_205384220_220000/RConn3 -- T_97872423__/LConn3 -- bus56/LConn1
  _CN_208263464_220000_CN_228718321_220000/RConn1 -- T_208263464__/LConn1 -- _CN_208263464_220000_CN_204983664_220000/LConn1
  _CN_208263464_220000_CN_228718321_220000/RConn2 -- T_208263464__/LConn2 -- _CN_208263464_220000_CN_204983664_220000/LConn2
  _CN_208263464_220000_CN_228718321_220000/RConn3 -- T_208263464__/LConn3 -- _CN_208263464_220000_CN_204983664_220000/LConn3 -- bus57/LConn1
  T_204983664__/LConn1 -- _CN_208263464_220000_CN_204983664_220000/RConn1
  T_204983664__/LConn2 -- _CN_208263464_220000_CN_204983664_220000/RConn2
  _CN_208263464_220000_CN_204983664_220000/RConn3 -- T_204983664__/LConn3 -- bus58/LConn1
  T_206558254__/LConn1 -- _CN_206558254_220000_CN_196654321_220000/LConn1
  T_206558254__/LConn2 -- _CN_206558254_220000_CN_196654321_220000/LConn2
  _CN_206558254_220000_CN_196654321_220000/LConn3 -- T_206558254__/LConn3 -- bus59/LConn1
  _CN_206558254_220000_CN_196654321_220000/RConn1 -- T_196654321__/RConn1 -- L_196654321/LConn1
  _CN_206558254_220000_CN_196654321_220000/RConn2 -- T_196654321__/RConn2 -- L_196654321/LConn2
  _CN_206558254_220000_CN_196654321_220000/RConn3 -- T_196654321__/RConn3 -- L_196654321/LConn3 -- bus60/LConn1
  _CN_288600947_220000_CN_199657972_220000/LConn1 -- T_288600947__Rovinari/RConn1 -- L_288600947/LConn1
  _CN_288600947_220000_CN_199657972_220000/LConn2 -- T_288600947__Rovinari/RConn2 -- L_288600947/LConn2
  _CN_288600947_220000_CN_199657972_220000/LConn3 -- T_288600947__Rovinari/RConn3 -- L_288600947/LConn3 -- bus61/LConn1
  _CN_288600947_220000_CN_199657972_220000/RConn1 -- T_199657972__/RConn1 -- L_199657972/LConn1
  _CN_288600947_220000_CN_199657972_220000/RConn2 -- T_199657972__/RConn2 -- L_199657972/LConn2
  _CN_288600947_220000_CN_199657972_220000/RConn3 -- T_199657972__/RConn3 -- L_199657972/LConn3 -- bus62/LConn1
  T_198901559__/LConn1 -- _CN_198901559_220000_CN_71212865_220000/LConn1
  T_198901559__/LConn2 -- _CN_198901559_220000_CN_71212865_220000/LConn2
  _CN_198901559_220000_CN_71212865_220000/LConn3 -- T_198901559__/LConn3 -- bus63/LConn1
  _CN_198901559_220000_CN_71212865_220000/RConn1 -- T_71212865__/LConn1 -- _CN_71212865_220000_CN_88174437_220000/RConn1
  _CN_198901559_220000_CN_71212865_220000/RConn2 -- T_71212865__/LConn2 -- _CN_71212865_220000_CN_88174437_220000/RConn2
  _CN_198901559_220000_CN_71212865_220000/RConn3 -- T_71212865__/LConn3 -- _CN_71212865_220000_CN_88174437_220000/RConn3 -- bus64/LConn1
  _CN_200720497_220000_CN_172029146_220000/LConn1 -- T_200720497__/LConn1 -- _CN_200720497_220000_CN_182655738_220000/LConn1
  _CN_200720497_220000_CN_172029146_220000/LConn2 -- T_200720497__/LConn2 -- _CN_200720497_220000_CN_182655738_220000/LConn2
  _CN_200720497_220000_CN_172029146_220000/LConn3 -- T_200720497__/LConn3 -- _CN_200720497_220000_CN_182655738_220000/LConn3 -- bus65/LConn1
  _CN_200720497_220000_CN_172029146_220000/RConn1 -- T_172029146__/LConn1 -- _CN_267616969_220000_CN_172029146_220000/LConn1
  _CN_200720497_220000_CN_172029146_220000/RConn2 -- T_172029146__/LConn2 -- _CN_267616969_220000_CN_172029146_220000/LConn2
  _CN_200720497_220000_CN_172029146_220000/RConn3 -- T_172029146__/LConn3 -- _CN_267616969_220000_CN_172029146_220000/LConn3 -- bus66/LConn1
  _CN_200720497_220000_CN_182655738_220000/RConn1 -- T_182655738__/RConn1 -- _CN_184476519_220000_CN_182655738_220000/LConn1 -- L_182655738/LConn1
  _CN_200720497_220000_CN_182655738_220000/RConn2 -- T_182655738__/RConn2 -- _CN_184476519_220000_CN_182655738_220000/LConn2 -- L_182655738/LConn2
  _CN_200720497_220000_CN_182655738_220000/RConn3 -- T_182655738__/RConn3 -- _CN_184476519_220000_CN_182655738_220000/LConn3 -- L_182655738/LConn3 -- bus67/LConn1
  T_267616969__/LConn1 -- _CN_267616969_220000_CN_172029146_220000/RConn1
  T_267616969__/LConn2 -- _CN_267616969_220000_CN_172029146_220000/RConn2
  _CN_267616969_220000_CN_172029146_220000/RConn3 -- T_267616969__/LConn3 -- bus68/LConn1
  T_184476519__/LConn1 -- _CN_184476519_220000_CN_182655738_220000/RConn1
  T_184476519__/LConn2 -- _CN_184476519_220000_CN_182655738_220000/RConn2
  _CN_184476519_220000_CN_182655738_220000/RConn3 -- T_184476519__/LConn3 -- bus69/LConn1
  T_208872170__/LConn1 -- _CN_208872170_220000_CN_101158766_220000/LConn1
  T_208872170__/LConn2 -- _CN_208872170_220000_CN_101158766_220000/LConn2
  _CN_208872170_220000_CN_101158766_220000/LConn3 -- T_208872170__/LConn3 -- bus70/LConn1
  _CN_208872170_220000_CN_101158766_220000/RConn1 -- T_101158766__/RConn1 -- L_101158766/LConn1
  _CN_208872170_220000_CN_101158766_220000/RConn2 -- T_101158766__/RConn2 -- L_101158766/LConn2
  _CN_208872170_220000_CN_101158766_220000/RConn3 -- T_101158766__/RConn3 -- L_101158766/LConn3 -- bus71/LConn1
  G_266629200_Electrica/RConn1 -- _CN_97334781_220000_CN_266629200_220000/RConn1
  G_266629200_Electrica/RConn2 -- _CN_97334781_220000_CN_266629200_220000/RConn2
  _CN_97334781_220000_CN_266629200_220000/RConn3 -- G_266629200_Electrica/RConn3 -- bus72/LConn1
  _CN_57888909_400000_CN_198777633_400000/LConn1 -- T_57888909__/LConn1 -- _CN_57888909_400000_CN_23575521_400000/LConn1
  _CN_57888909_400000_CN_198777633_400000/LConn2 -- T_57888909__/LConn2 -- _CN_57888909_400000_CN_23575521_400000/LConn2
  _CN_57888909_400000_CN_198777633_400000/LConn3 -- T_57888909__/LConn3 -- _CN_57888909_400000_CN_23575521_400000/LConn3 -- bus73/LConn1
  _CN_57888909_400000_CN_198777633_400000/RConn1 -- T_198777633__/LConn1 -- _CN_198777633_400000_CN_228718321_400000/LConn1 -- _CN_198777633_400000_CN_196654321_400000/LConn1 -- _CN_198777633_400000_CN_204969810_400000/LConn1
  _CN_57888909_400000_CN_198777633_400000/RConn2 -- T_198777633__/LConn2 -- _CN_198777633_400000_CN_228718321_400000/LConn2 -- _CN_198777633_400000_CN_196654321_400000/LConn2 -- _CN_198777633_400000_CN_204969810_400000/LConn2
  _CN_57888909_400000_CN_198777633_400000/RConn3 -- T_198777633__/LConn3 -- _CN_198777633_400000_CN_228718321_400000/LConn3 -- _CN_198777633_400000_CN_196654321_400000/LConn3 -- _CN_198777633_400000_CN_204969810_400000/LConn3 -- bus74/LConn1
  _CN_57888909_400000_CN_23575521_400000/RConn1 -- T_23575521__/LConn1 -- Linie_electrică_de_înaltă_tensiune_de_400_kV_CN_28251692_400000_CN_23575521_400000/LConn1 -- _CN_232578495_400000_CN_23575521_400000/LConn1
  _CN_57888909_400000_CN_23575521_400000/RConn2 -- T_23575521__/LConn2 -- Linie_electrică_de_înaltă_tensiune_de_400_kV_CN_28251692_400000_CN_23575521_400000/LConn2 -- _CN_232578495_400000_CN_23575521_400000/LConn2
  _CN_57888909_400000_CN_23575521_400000/RConn3 -- T_23575521__/LConn3 -- Linie_electrică_de_înaltă_tensiune_de_400_kV_CN_28251692_400000_CN_23575521_400000/LConn3 -- _CN_232578495_400000_CN_23575521_400000/LConn3 -- bus75/LConn1
  T_196672685__/LConn1 -- _CN_196672685_400000_CN_196672665_400000/LConn1
  T_196672685__/LConn2 -- _CN_196672685_400000_CN_196672665_400000/LConn2
  _CN_196672685_400000_CN_196672665_400000/LConn3 -- T_196672685__/LConn3 -- bus76/LConn1
  _CN_196672685_400000_CN_196672665_400000/RConn1 -- T_196672665__/LConn1 -- _CN_196672665_400000_CN_232578495_400000/LConn1 -- _CN_196672665_400000_CN_125672002_400000/LConn1
  _CN_196672685_400000_CN_196672665_400000/RConn2 -- T_196672665__/LConn2 -- _CN_196672665_400000_CN_232578495_400000/LConn2 -- _CN_196672665_400000_CN_125672002_400000/LConn2
  _CN_196672685_400000_CN_196672665_400000/RConn3 -- T_196672665__/LConn3 -- _CN_196672665_400000_CN_232578495_400000/LConn3 -- _CN_196672665_400000_CN_125672002_400000/LConn3 -- bus77/LConn1
  T_234876688__/LConn1 -- _CN_234876688_400000_CN_202948507_400000/LConn1
  T_234876688__/LConn2 -- _CN_234876688_400000_CN_202948507_400000/LConn2
  _CN_234876688_400000_CN_202948507_400000/LConn3 -- T_234876688__/LConn3 -- bus78/LConn1
  T_202948507__/LConn1 -- _CN_234876688_400000_CN_202948507_400000/RConn1
  T_202948507__/LConn2 -- _CN_234876688_400000_CN_202948507_400000/RConn2
  _CN_234876688_400000_CN_202948507_400000/RConn3 -- T_202948507__/LConn3 -- bus79/LConn1
  _CN_234876695_400000_CN_196557387_400000/LConn1 -- T_234876695__/LConn1 -- _CN_234876695_400000_CN_196654321_400000/LConn1
  _CN_234876695_400000_CN_196557387_400000/LConn2 -- T_234876695__/LConn2 -- _CN_234876695_400000_CN_196654321_400000/LConn2
  _CN_234876695_400000_CN_196557387_400000/LConn3 -- T_234876695__/LConn3 -- _CN_234876695_400000_CN_196654321_400000/LConn3 -- bus80/LConn1
  _CN_234876695_400000_CN_196557387_400000/RConn1 -- T_196557387__/LConn1 -- _CN_205252518_400000_CN_196557387_400000/LConn1
  _CN_234876695_400000_CN_196557387_400000/RConn2 -- T_196557387__/LConn2 -- _CN_205252518_400000_CN_196557387_400000/LConn2
  _CN_234876695_400000_CN_196557387_400000/RConn3 -- T_196557387__/LConn3 -- _CN_205252518_400000_CN_196557387_400000/LConn3 -- bus81/LConn1
  _CN_234876695_400000_CN_196654321_400000/RConn1 -- T_196654321__/LConn1 -- _CN_196654321_400000_CN_88174437_220000/RConn1 -- _CN_205384220_400000_CN_196654321_400000/LConn1 -- _CN_198777633_400000_CN_196654321_400000/RConn1
  _CN_234876695_400000_CN_196654321_400000/RConn2 -- T_196654321__/LConn2 -- _CN_196654321_400000_CN_88174437_220000/RConn2 -- _CN_205384220_400000_CN_196654321_400000/LConn2 -- _CN_198777633_400000_CN_196654321_400000/RConn2
  _CN_234876695_400000_CN_196654321_400000/RConn3 -- T_196654321__/LConn3 -- _CN_196654321_400000_CN_88174437_220000/RConn3 -- bus82/LConn1 -- _CN_205384220_400000_CN_196654321_400000/LConn3 -- _CN_198777633_400000_CN_196654321_400000/RConn3
  _CN_196672665_400000_CN_232578495_400000/RConn1 -- T_232578495__/LConn1 -- _CN_232578495_400000_CN_23575521_400000/RConn1
  _CN_196672665_400000_CN_232578495_400000/RConn2 -- T_232578495__/LConn2 -- _CN_232578495_400000_CN_23575521_400000/RConn2
  _CN_196672665_400000_CN_232578495_400000/RConn3 -- T_232578495__/LConn3 -- _CN_232578495_400000_CN_23575521_400000/RConn3 -- bus83/LConn1
  T_125672002__/LConn1 -- _CN_196672665_400000_CN_125672002_400000/RConn1
  T_125672002__/LConn2 -- _CN_196672665_400000_CN_125672002_400000/RConn2
  _CN_196672665_400000_CN_125672002_400000/RConn3 -- T_125672002__/LConn3 -- bus84/LConn1
  _CN_205384220_400000_CN_196654321_400000/RConn1 -- T_205384220__/LConn1 -- _CN_205384220_400000_CN_199657972_400000/LConn1
  _CN_205384220_400000_CN_196654321_400000/RConn2 -- T_205384220__/LConn2 -- _CN_205384220_400000_CN_199657972_400000/LConn2
  _CN_205384220_400000_CN_196654321_400000/RConn3 -- T_205384220__/LConn3 -- _CN_205384220_400000_CN_199657972_400000/LConn3 -- bus85/LConn1
  _CN_205384220_400000_CN_199657972_400000/RConn1 -- T_199657972__/LConn1 -- _CN_28251692_400000_CN_199657972_400000/LConn1 -- _CN_288600947_400000_CN_199657972_400000/LConn1 -- _CN_228718321_400000_CN_199657972_400000/LConn1
  _CN_205384220_400000_CN_199657972_400000/RConn2 -- T_199657972__/LConn2 -- _CN_28251692_400000_CN_199657972_400000/LConn2 -- _CN_288600947_400000_CN_199657972_400000/LConn2 -- _CN_228718321_400000_CN_199657972_400000/LConn2
  _CN_205384220_400000_CN_199657972_400000/RConn3 -- T_199657972__/LConn3 -- _CN_28251692_400000_CN_199657972_400000/LConn3 -- _CN_288600947_400000_CN_199657972_400000/LConn3 -- bus86/LConn1 -- _CN_228718321_400000_CN_199657972_400000/LConn3
  _CN_198777633_400000_CN_228718321_400000/RConn1 -- T_228718321__/LConn1 -- _CN_228718321_400000_CN_199657972_400000/RConn1 -- _CN_228718321_400000_CN_238952272_400000/LConn1
  _CN_198777633_400000_CN_228718321_400000/RConn2 -- T_228718321__/LConn2 -- _CN_228718321_400000_CN_199657972_400000/RConn2 -- _CN_228718321_400000_CN_238952272_400000/LConn2
  _CN_198777633_400000_CN_228718321_400000/RConn3 -- T_228718321__/LConn3 -- _CN_228718321_400000_CN_199657972_400000/RConn3 -- _CN_228718321_400000_CN_238952272_400000/LConn3 -- bus87/LConn1
  T_204969810__/LConn1 -- _CN_198777633_400000_CN_204969810_400000/RConn1
  T_204969810__/LConn2 -- _CN_198777633_400000_CN_204969810_400000/RConn2
  _CN_198777633_400000_CN_204969810_400000/RConn3 -- T_204969810__/LConn3 -- bus88/LConn1
  T_205252518__Statia_Cluj_Est/LConn1 -- _CN_205252518_400000_CN_196557387_400000/RConn1
  T_205252518__Statia_Cluj_Est/LConn2 -- _CN_205252518_400000_CN_196557387_400000/RConn2
  _CN_205252518_400000_CN_196557387_400000/RConn3 -- T_205252518__Statia_Cluj_Est/LConn3 -- bus89/LConn1
  _CN_228718321_400000_CN_238952272_400000/RConn1 -- T_238952272__/LConn1 -- _CN_238952272_400000_CN_342979123_400000/LConn1
  _CN_228718321_400000_CN_238952272_400000/RConn2 -- T_238952272__/LConn2 -- _CN_238952272_400000_CN_342979123_400000/LConn2
  _CN_228718321_400000_CN_238952272_400000/RConn3 -- T_238952272__/LConn3 -- _CN_238952272_400000_CN_342979123_400000/LConn3 -- bus90/LConn1
  Békéscsaba–Nagyvárad_távvezeték_CN_195155625_400000_CN_195168461_400000/LConn1 -- T_195155625__/LConn1 -- _CN_195155625_400000_CN_101158766_400000/LConn1
  Békéscsaba–Nagyvárad_távvezeték_CN_195155625_400000_CN_195168461_400000/LConn2 -- T_195155625__/LConn2 -- _CN_195155625_400000_CN_101158766_400000/LConn2
  Békéscsaba–Nagyvárad_távvezeték_CN_195155625_400000_CN_195168461_400000/LConn3 -- T_195155625__/LConn3 -- _CN_195155625_400000_CN_101158766_400000/LConn3 -- bus91/LConn1
  T_195168461__/LConn1 -- Békéscsaba–Nagyvárad_távvezeték_CN_195155625_400000_CN_195168461_400000/RConn1
  T_195168461__/LConn2 -- Békéscsaba–Nagyvárad_távvezeték_CN_195155625_400000_CN_195168461_400000/RConn2
  Békéscsaba–Nagyvárad_távvezeték_CN_195155625_400000_CN_195168461_400000/RConn3 -- T_195168461__/LConn3 -- bus92/LConn1
  _CN_195155625_400000_CN_101158766_400000/RConn1 -- T_101158766__/LConn1 -- _CN_101158766_400000_CN_88174437_220000/RConn1
  _CN_195155625_400000_CN_101158766_400000/RConn2 -- T_101158766__/LConn2 -- _CN_101158766_400000_CN_88174437_220000/RConn2
  _CN_195155625_400000_CN_101158766_400000/RConn3 -- T_101158766__/LConn3 -- _CN_101158766_400000_CN_88174437_220000/RConn3 -- bus93/LConn1
  _CN_28251692_400000_CN_199657972_400000/RConn1 -- T_28251692__/LConn1 -- Linie_electrică_de_înaltă_tensiune_de_400_kV_CN_28251692_400000_CN_23575521_400000/RConn1 -- _CN_28251692_400000_CN_198333299_400000/LConn1
  _CN_28251692_400000_CN_199657972_400000/RConn2 -- T_28251692__/LConn2 -- Linie_electrică_de_înaltă_tensiune_de_400_kV_CN_28251692_400000_CN_23575521_400000/RConn2 -- _CN_28251692_400000_CN_198333299_400000/LConn2
  _CN_28251692_400000_CN_199657972_400000/RConn3 -- T_28251692__/LConn3 -- Linie_electrică_de_înaltă_tensiune_de_400_kV_CN_28251692_400000_CN_23575521_400000/RConn3 -- bus94/LConn1 -- _CN_28251692_400000_CN_198333299_400000/LConn3
  T_198333299__/LConn1 -- _CN_28251692_400000_CN_198333299_400000/RConn1
  T_198333299__/LConn2 -- _CN_28251692_400000_CN_198333299_400000/RConn2
  _CN_28251692_400000_CN_198333299_400000/RConn3 -- T_198333299__/LConn3 -- bus95/LConn1
  T_288600947__Rovinari/LConn1 -- _CN_288600947_400000_CN_199657972_400000/RConn1
  T_288600947__Rovinari/LConn2 -- _CN_288600947_400000_CN_199657972_400000/RConn2
  _CN_288600947_400000_CN_199657972_400000/RConn3 -- T_288600947__Rovinari/LConn3 -- bus96/LConn1
  T_191363648__/LConn1 -- _CN_191363648_400000_CN_182655738_400000/LConn1
  T_191363648__/LConn2 -- _CN_191363648_400000_CN_182655738_400000/LConn2
  _CN_191363648_400000_CN_182655738_400000/LConn3 -- T_191363648__/LConn3 -- bus97/LConn1
  T_182655738__/LConn1 -- _CN_191363648_400000_CN_182655738_400000/RConn1
  T_182655738__/LConn2 -- _CN_191363648_400000_CN_182655738_400000/RConn2
  _CN_191363648_400000_CN_182655738_400000/RConn3 -- T_182655738__/LConn3 -- bus98/LConn1
  G_342979123_Хидроелектрана_Ђердап_I/RConn1 -- _CN_238952272_400000_CN_342979123_400000/RConn1
  G_342979123_Хидроелектрана_Ђердап_I/RConn2 -- _CN_238952272_400000_CN_342979123_400000/RConn2
  _CN_238952272_400000_CN_342979123_400000/RConn3 -- G_342979123_Хидроелектрана_Ђердап_I/RConn3 -- bus99/LConn1
  T_48374400__/RConn1 -- L_48374400/LConn1
  T_48374400__/RConn2 -- L_48374400/LConn2
  L_48374400/LConn3 -- T_48374400__/RConn3 -- bus100/LConn1
  T_46584322__/RConn1 -- L_46584322/LConn1
  T_46584322__/RConn2 -- L_46584322/LConn2
  L_46584322/LConn3 -- T_46584322__/RConn3 -- bus101/LConn1
  T_209067396__/RConn1 -- L_209067396/LConn1
  T_209067396__/RConn2 -- L_209067396/LConn2
  L_209067396/LConn3 -- T_209067396__/RConn3 -- bus102/LConn1
  T_30621843__/RConn1 -- L_30621843/LConn1
  T_30621843__/RConn2 -- L_30621843/LConn2
  L_30621843/LConn3 -- T_30621843__/RConn3 -- bus103/LConn1
  T_30622639__/RConn1 -- L_30622639/LConn1
  T_30622639__/RConn2 -- L_30622639/LConn2
  L_30622639/LConn3 -- T_30622639__/RConn3 -- bus104/LConn1
  T_207939980__/RConn1 -- L_207939980/LConn1
  T_207939980__/RConn2 -- L_207939980/LConn2
  L_207939980/LConn3 -- T_207939980__/RConn3 -- bus105/LConn1
  T_176819478__Statie_de_transformare_110kV_20kV/RConn1 -- L_176819478/LConn1
  T_176819478__Statie_de_transformare_110kV_20kV/RConn2 -- L_176819478/LConn2
  L_176819478/LConn3 -- T_176819478__Statie_de_transformare_110kV_20kV/RConn3 -- bus106/LConn1
  T_97418808__/RConn1 -- L_97418808/LConn1
  T_97418808__/RConn2 -- L_97418808/LConn2
  L_97418808/LConn3 -- T_97418808__/RConn3 -- bus107/LConn1
  T_204932122__/RConn1 -- L_204932122/LConn1
  T_204932122__/RConn2 -- L_204932122/LConn2
  L_204932122/LConn3 -- T_204932122__/RConn3 -- bus108/LConn1
  T_198333274__/RConn1 -- L_198333274/LConn1
  T_198333274__/RConn2 -- L_198333274/LConn2
  L_198333274/LConn3 -- T_198333274__/RConn3 -- bus109/LConn1
  T_97334822__/RConn1 -- L_97334822/LConn1
  T_97334822__/RConn2 -- L_97334822/LConn2
  L_97334822/LConn3 -- T_97334822__/RConn3 -- bus110/LConn1
  T_37036252__/RConn1 -- L_37036252/LConn1
  T_37036252__/RConn2 -- L_37036252/LConn2
  L_37036252/LConn3 -- T_37036252__/RConn3 -- bus111/LConn1
  T_176828096__/RConn1 -- L_176828096/LConn1
  T_176828096__/RConn2 -- L_176828096/LConn2
  L_176828096/LConn3 -- T_176828096__/RConn3 -- bus112/LConn1
  T_235313249__/RConn1 -- L_235313249/LConn1
  T_235313249__/RConn2 -- L_235313249/LConn2
  L_235313249/LConn3 -- T_235313249__/RConn3 -- bus113/LConn1
  T_29975403__/RConn1 -- L_29975403/LConn1
  T_29975403__/RConn2 -- L_29975403/LConn2
  L_29975403/LConn3 -- T_29975403__/RConn3 -- bus114/LConn1
  T_89071477__/RConn1 -- L_89071477/LConn1
  T_89071477__/RConn2 -- L_89071477/LConn2
  L_89071477/LConn3 -- T_89071477__/RConn3 -- bus115/LConn1
  T_46269303__/RConn1 -- L_46269303/LConn1
  T_46269303__/RConn2 -- L_46269303/LConn2
  L_46269303/LConn3 -- T_46269303__/RConn3 -- bus116/LConn1
  T_278910976__/RConn1 -- L_278910976/LConn1
  T_278910976__/RConn2 -- L_278910976/LConn2
  L_278910976/LConn3 -- T_278910976__/RConn3 -- bus117/LConn1
  T_199657993__/RConn1 -- L_199657993/LConn1
  T_199657993__/RConn2 -- L_199657993/LConn2
  L_199657993/LConn3 -- T_199657993__/RConn3 -- bus118/LConn1
  T_208744453__/RConn1 -- L_208744453/LConn1
  T_208744453__/RConn2 -- L_208744453/LConn2
  L_208744453/LConn3 -- T_208744453__/RConn3 -- bus119/LConn1
  T_198276673__/RConn1 -- L_198276673/LConn1
  T_198276673__/RConn2 -- L_198276673/LConn2
  L_198276673/LConn3 -- T_198276673__/RConn3 -- bus120/LConn1
  T_202461729__/RConn1 -- L_202461729/LConn1
  T_202461729__/RConn2 -- L_202461729/LConn2
  L_202461729/LConn3 -- T_202461729__/RConn3 -- bus121/LConn1
  T_98111242__/RConn1 -- L_98111242/LConn1
  T_98111242__/RConn2 -- L_98111242/LConn2
  L_98111242/LConn3 -- T_98111242__/RConn3 -- bus122/LConn1
  T_196654384__/RConn1 -- L_196654384/LConn1
  T_196654384__/RConn2 -- L_196654384/LConn2
  L_196654384/LConn3 -- T_196654384__/RConn3 -- bus123/LConn1
  T_208263479__/RConn1 -- L_208263479/LConn1
  T_208263479__/RConn2 -- L_208263479/LConn2
  L_208263479/LConn3 -- T_208263479__/RConn3 -- bus124/LConn1
  T_198283094__/RConn1 -- L_198283094/LConn1
  T_198283094__/RConn2 -- L_198283094/LConn2
  L_198283094/LConn3 -- T_198283094__/RConn3 -- bus125/LConn1
  T_196654364__/RConn1 -- L_196654364/LConn1
  T_196654364__/RConn2 -- L_196654364/LConn2
  L_196654364/LConn3 -- T_196654364__/RConn3 -- bus126/LConn1
  T_196654362__/RConn1 -- L_196654362/LConn1
  T_196654362__/RConn2 -- L_196654362/LConn2
  L_196654362/LConn3 -- T_196654362__/RConn3 -- bus127/LConn1
  T_108198802__/RConn1 -- L_108198802/LConn1
  T_108198802__/RConn2 -- L_108198802/LConn2
  L_108198802/LConn3 -- T_108198802__/RConn3 -- bus128/LConn1
  T_108198777__/RConn1 -- L_108198777/LConn1
  T_108198777__/RConn2 -- L_108198777/LConn2
  L_108198777/LConn3 -- T_108198777__/RConn3 -- bus129/LConn1
  T_30621463__/RConn1 -- L_30621463/LConn1
  T_30621463__/RConn2 -- L_30621463/LConn2
  L_30621463/LConn3 -- T_30621463__/RConn3 -- bus130/LConn1
  T_198310955__/RConn1 -- L_198310955/LConn1
  T_198310955__/RConn2 -- L_198310955/LConn2
  L_198310955/LConn3 -- T_198310955__/RConn3 -- bus131/LConn1
  T_210609562__/RConn1 -- L_210609562/LConn1
  T_210609562__/RConn2 -- L_210609562/LConn2
  L_210609562/LConn3 -- T_210609562__/RConn3 -- bus132/LConn1
  T_208294493__/RConn1 -- L_208294493/LConn1
  T_208294493__/RConn2 -- L_208294493/LConn2
  L_208294493/LConn3 -- T_208294493__/RConn3 -- bus133/LConn1
  T_223680127__/RConn1 -- L_223680127/LConn1
  T_223680127__/RConn2 -- L_223680127/LConn2
  L_223680127/LConn3 -- T_223680127__/RConn3 -- bus134/LConn1
  T_198777681__/RConn1 -- L_198777681/LConn1
  T_198777681__/RConn2 -- L_198777681/LConn2
  L_198777681/LConn3 -- T_198777681__/RConn3 -- bus135/LConn1
  T_103213478__/RConn1 -- L_103213478/LConn1
  T_103213478__/RConn2 -- L_103213478/LConn2
  L_103213478/LConn3 -- T_103213478__/RConn3 -- bus136/LConn1
  T_182886368__/RConn1 -- L_182886368/LConn1
  T_182886368__/RConn2 -- L_182886368/LConn2
  L_182886368/LConn3 -- T_182886368__/RConn3 -- bus137/LConn1
  T_74348980__/RConn1 -- L_74348980/LConn1
  T_74348980__/RConn2 -- L_74348980/LConn2
  L_74348980/LConn3 -- T_74348980__/RConn3 -- bus138/LConn1
  T_97872423__/RConn1 -- L_97872423/LConn1
  T_97872423__/RConn2 -- L_97872423/LConn2
  L_97872423/LConn3 -- T_97872423__/RConn3 -- bus139/LConn1
  T_208263464__/RConn1 -- L_208263464/LConn1
  T_208263464__/RConn2 -- L_208263464/LConn2
  L_208263464/LConn3 -- T_208263464__/RConn3 -- bus140/LConn1
  T_204983664__/RConn1 -- L_204983664/LConn1
  T_204983664__/RConn2 -- L_204983664/LConn2
  L_204983664/LConn3 -- T_204983664__/RConn3 -- bus141/LConn1
  T_206558254__/RConn1 -- L_206558254/LConn1
  T_206558254__/RConn2 -- L_206558254/LConn2
  L_206558254/LConn3 -- T_206558254__/RConn3 -- bus142/LConn1
  T_198901559__/RConn1 -- L_198901559/LConn1
  T_198901559__/RConn2 -- L_198901559/LConn2
  L_198901559/LConn3 -- T_198901559__/RConn3 -- bus143/LConn1
  T_71212865__/RConn1 -- L_71212865/LConn1
  T_71212865__/RConn2 -- L_71212865/LConn2
  L_71212865/LConn3 -- T_71212865__/RConn3 -- bus144/LConn1
  T_200720497__/RConn1 -- L_200720497/LConn1
  T_200720497__/RConn2 -- L_200720497/LConn2
  L_200720497/LConn3 -- T_200720497__/RConn3 -- bus145/LConn1
  T_172029146__/RConn1 -- L_172029146/LConn1
  T_172029146__/RConn2 -- L_172029146/LConn2
  L_172029146/LConn3 -- T_172029146__/RConn3 -- bus146/LConn1
  T_267616969__/RConn1 -- L_267616969/LConn1
  T_267616969__/RConn2 -- L_267616969/LConn2
  L_267616969/LConn3 -- T_267616969__/RConn3 -- bus147/LConn1
  T_184476519__/RConn1 -- L_184476519/LConn1
  T_184476519__/RConn2 -- L_184476519/LConn2
  L_184476519/LConn3 -- T_184476519__/RConn3 -- bus148/LConn1
  T_208872170__/RConn1 -- L_208872170/LConn1
  T_208872170__/RConn2 -- L_208872170/LConn2
  L_208872170/LConn3 -- T_208872170__/RConn3 -- bus149/LConn1
  T_57888909__/RConn1 -- L_57888909/LConn1
  T_57888909__/RConn2 -- L_57888909/LConn2
  L_57888909/LConn3 -- T_57888909__/RConn3 -- bus150/LConn1
  T_234876688__/RConn1 -- L_234876688/LConn1
  T_234876688__/RConn2 -- L_234876688/LConn2
  L_234876688/LConn3 -- T_234876688__/RConn3 -- bus151/LConn1
  T_196557387__/RConn1 -- L_196557387/LConn1
  T_196557387__/RConn2 -- L_196557387/LConn2
  L_196557387/LConn3 -- T_196557387__/RConn3 -- bus152/LConn1
  T_232578495__/RConn1 -- L_232578495/LConn1
  T_232578495__/RConn2 -- L_232578495/LConn2
  L_232578495/LConn3 -- T_232578495__/RConn3 -- bus153/LConn1
  T_125672002__/RConn1 -- L_125672002/LConn1
  T_125672002__/RConn2 -- L_125672002/LConn2
  L_125672002/LConn3 -- T_125672002__/RConn3 -- bus154/LConn1
  T_204969810__/RConn1 -- L_204969810/LConn1
  T_204969810__/RConn2 -- L_204969810/LConn2
  L_204969810/LConn3 -- T_204969810__/RConn3 -- bus155/LConn1
  T_205252518__Statia_Cluj_Est/RConn1 -- L_205252518/LConn1
  T_205252518__Statia_Cluj_Est/RConn2 -- L_205252518/LConn2
  L_205252518/LConn3 -- T_205252518__Statia_Cluj_Est/RConn3 -- bus156/LConn1
  T_238952272__/RConn1 -- L_238952272/LConn1
  T_238952272__/RConn2 -- L_238952272/LConn2
  L_238952272/LConn3 -- T_238952272__/RConn3 -- bus157/LConn1
  T_195155625__/RConn1 -- L_195155625/LConn1
  T_195155625__/RConn2 -- L_195155625/LConn2
  L_195155625/LConn3 -- T_195155625__/RConn3 -- bus158/LConn1
  T_195168461__/RConn1 -- L_195168461/LConn1
  T_195168461__/RConn2 -- L_195168461/LConn2
  L_195168461/LConn3 -- T_195168461__/RConn3 -- bus159/LConn1
  T_198333299__/RConn1 -- L_198333299/LConn1
  T_198333299__/RConn2 -- L_198333299/LConn2
  L_198333299/LConn3 -- T_198333299__/RConn3 -- bus160/LConn1
  T_191363648__/RConn1 -- L_191363648/LConn1
  T_191363648__/RConn2 -- L_191363648/LConn2
  L_191363648/LConn3 -- T_191363648__/RConn3 -- bus161/LConn1
